simulink model "masterRobotAndOperator_v2"  (R2021b)
settings: Solver=VariableStepAuto  StartTime=0.0  StopTime=10  RelTol=1e-3
undefined symbols (not defined in the file): A, Bh, Dh, Fc, Flp, Jh, Mm, Ph
settings Model: Creator=riccardo  LastModifiedBy=riccardo

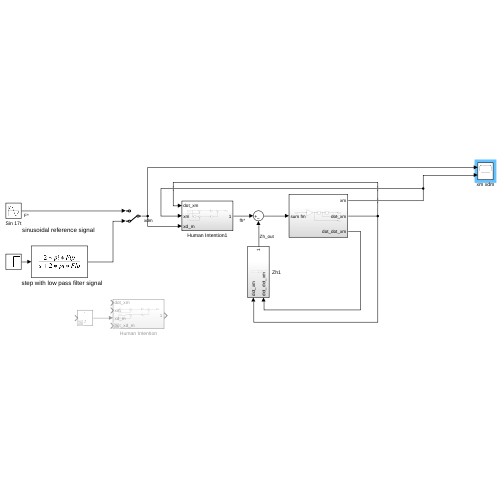
[thumbnail: Simulink's stored preview of the top-level diagram]
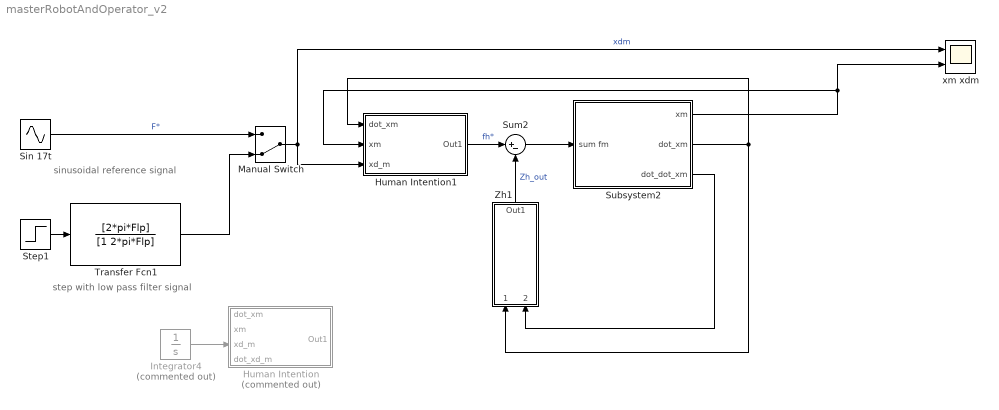
== system masterRobotAndOperator_v2 ==
  note: step with low pass filter signal
  note: sinusoidal reference signal
  Human Intention : Subsystem  Commented=on
  Human Intention1 : Subsystem
  Integrator4 : Integrator  Commented=on
  Manual Switch : ManualSwitch  CurrentSetting=0
  Sin 17t : Sin  Amplitude=A  Frequency=2*pi*Fc  SampleTime=0
  Step1 : Step  Time=0.5  After=A  SampleTime=0
  Subsystem2 : Subsystem
  Sum2 : Sum  Inputs=|+-
  Transfer Fcn1 : TransferFcn  Numerator=[2*pi*Flp]  Denominator=[1 2*pi*Flp]
  Zh1 : Subsystem
  xm xdm : Scope  NumInputPorts=2
  wires:
  Sum2/1 -> Subsystem2/1(sum fm)
  Subsystem2/1(xm) -> Human Intention1/2(xm), xm xdm/2
  Manual Switch/1 -> Human Intention1/3(xd_m), xm xdm/1  "xdm"
  Transfer Fcn1/1 -> Manual Switch/2
  Step1/1 -> Transfer Fcn1/1
  Zh1/1(Out1) -> Sum2/2  "Zh_out"
  Sin 17t/1 -> Manual Switch/1  "F*"
  Human Intention1/1(Out1) -> Sum2/1  "fh*"
  Subsystem2/3(dot_dot_xm) -> Zh1/2(dot_dot_xm)
  Subsystem2/2(dot_xm) -> Human Intention1/1(dot_xm), Zh1/1(dot_xm)
  Integrator4/1 -> Human Intention/3(xd_m)

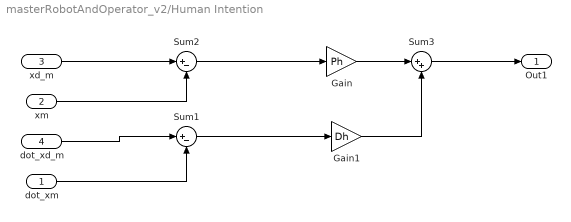
== system masterRobotAndOperator_v2/Human Intention ==
  dot_xm : Inport
  xm : Inport  Port=2
  xd_m : Inport  Port=3
  dot_xd_m : Inport  Port=4
  Gain : Gain  Gain=Ph
  Gain1 : Gain  Gain=Dh
  Sum1 : Sum  Inputs=|+-
  Sum2 : Sum  Inputs=|+-
  Sum3 : Sum  Inputs=|++
  Out1 : Outport
  wires:
  xm/1 -> Sum2/2
  dot_xm/1 -> Sum1/2
  Sum2/1 -> Gain/1
  Sum1/1 -> Gain1/1
  Gain1/1 -> Sum3/2
  Gain/1 -> Sum3/1
  xd_m/1 -> Sum2/1
  Sum3/1 -> Out1/1
  dot_xd_m/1 -> Sum1/1

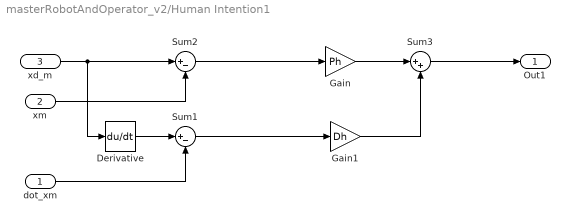
== system masterRobotAndOperator_v2/Human Intention1 ==
  dot_xm : Inport
  xm : Inport  Port=2
  xd_m : Inport  Port=3
  Derivative : Derivative
  Gain : Gain  Gain=Ph
  Gain1 : Gain  Gain=Dh
  Sum1 : Sum  Inputs=|+-
  Sum2 : Sum  Inputs=|+-
  Sum3 : Sum  Inputs=|++
  Out1 : Outport
  wires:
  xm/1 -> Sum2/2
  dot_xm/1 -> Sum1/2
  Sum2/1 -> Gain/1
  Sum1/1 -> Gain1/1
  Gain1/1 -> Sum3/2
  Gain/1 -> Sum3/1
  Sum3/1 -> Out1/1
  xd_m/1 -> Derivative/1, Sum2/1
  Derivative/1 -> Sum1/1

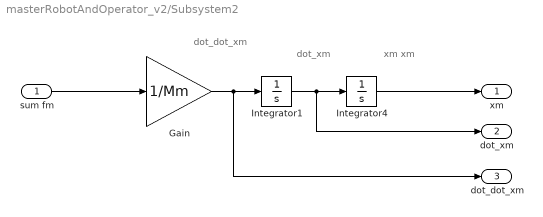
== system masterRobotAndOperator_v2/Subsystem2 ==
  note: dot_dot_xm
  note: dot_xm
  note: xm
      | xm
  sum fm : Inport
  Gain : Gain  Gain=1/Mm
  Integrator1 : Integrator
  Integrator4 : Integrator
  xm : Outport
  dot_xm : Outport  Port=2
  dot_dot_xm : Outport  Port=3
  wires:
  sum fm/1 -> Gain/1
  Gain/1 -> dot_dot_xm/1, Integrator1/1
  Integrator4/1 -> xm/1
  Integrator1/1 -> dot_xm/1, Integrator4/1

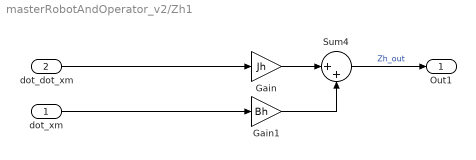
== system masterRobotAndOperator_v2/Zh1 ==
  dot_xm : Inport
  dot_dot_xm : Inport  Port=2
  Gain : Gain  Gain=Jh
  Gain1 : Gain  Gain=Bh
  Sum4 : Sum  Inputs=|++
  Out1 : Outport
  wires:
  dot_dot_xm/1 -> Gain/1
  Gain1/1 -> Sum4/2
  Gain/1 -> Sum4/1
  Sum4/1 -> Out1/1  "Zh_out"
  dot_xm/1 -> Gain1/1
